simulink model "MPPT"  (R2024a)
settings: Solver=VariableStepAuto  StartTime=0.0  StopTime=0.3  FixedStep=0.02  RelTol=1e-3
libraries: spsSeriesRLCBranchLib x4, spsDiodeLib x2, spsCurrentMeasurementLib x1, spsMosfetLib x1, spsPVArrayLib x1, spsPWMGeneratorDCDCLib x1, spsVoltageMeasurementLib x1, sps_lib x1
settings Model: Creator=ACER  LastModifiedBy=Aswathi Sajeev
settings SolverCC: AlgebraicLoopSolver=TrustRegion
settings DataIOCC: ReturnWorkspaceOutputs=off
settings DebuggingCC: UnconnectedInputMsg=warning  UnconnectedOutputMsg=warning  UnconnectedLineMsg=warning  ArithmeticOperatorsInVariantConditions=warning
settings ModelReferenceCC: EnableRefExpFcnMdlSchedulingChecks=on
settings SFSimCC: SimUseLocalCustomCode=off  CustomCodeUndefinedFunction=UseInterfaceOnly
settings RTWCC: RTWUseLocalCustomCode=off  GPUComputeCapability=3.5

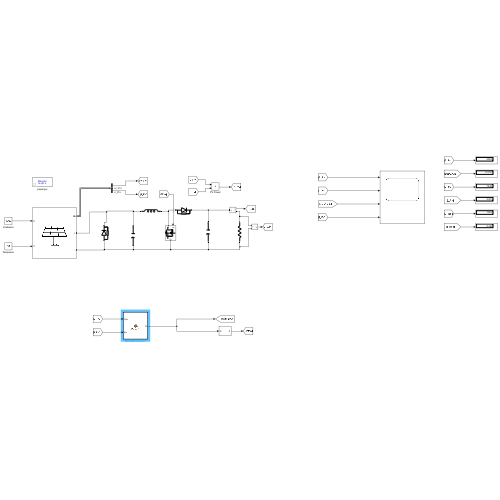
[thumbnail: Simulink's stored preview of the top-level diagram]
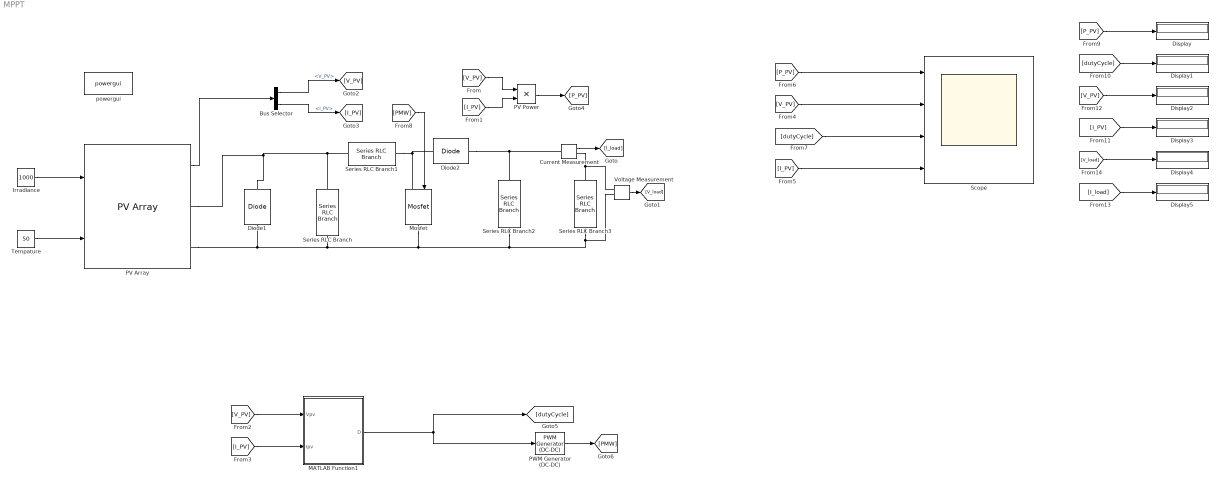
== system MPPT ==
  Bus Selector : BusSelector  OutputSignals=V_PV,I_PV
  Current Measurement : spsCurrentMeasurementLib/Current Measurement  PhasorSimulation=off  OutputType=Complex  PSBequivalent=0
  Diode1 : spsDiodeLib/Diode  Ron=0.001  Lon=0  Vf=0.8  IC=0  UseSnubber=0  Rs=500  Cs=250e-9  Measurements=off
  Diode2 : spsDiodeLib/Diode  Ron=0.001  Lon=0  Vf=0.8  IC=0  UseSnubber=0  Rs=500  Cs=250e-9  Measurements=off
  Display{,1..5} (6 alike) : Display
  Irradiance : Constant  Value=1000
  MATLAB Function1 : MATLAB Function  TreatAsAtomicUnit=on
  Mosfet : spsMosfetLib/Mosfet  Ron=1e-3  Lon=0  Rd=1e-3  Vfd=0  IC=0  Rs=inf  Cs=inf  Measurements=off
  PV Array : spsPVArrayLib/PV Array  Npar=1  Nser=6  PlotType=array @ 1000 W/m2 & specified temperatures  S_vec=[1000 800 400]  Temp_C_vec=[25 50 75]  ModuleName=User-defined  PlotWhenSelected=off  Pm=55.5  Ncell=36  Voc=21.7  Isc=4.8  Vm=15  Im=3.7  beta_Voc_pc=-0.33641  alpha_Isc_pc=0.102  beta_Voc=-0.073001  alpha_Isc=0.004896  IL=5.1461  I0=7.3617e-11  nI=0.95111  Rsh=16.138  Rs=1.1636  RobustModel=off  RobustCellTemperature=313.3991  BAL=off  Tc=1e-6  Tfilter=5e-5
  PV Power : Product
  PWM Generator (DC-DC) : spsPWMGeneratorDCDCLib/PWM Generator (DC-DC)  Fsw=10000  Ts=10e-6
  Scope : Scope  NumInputPorts=4
  Series RLC Branch : spsSeriesRLCBranchLib/Series RLC Branch  LConnTagsString=__new0  RConnTagsString=__new0  BranchType=C  Resistance=1  Inductance=1e-3  SetiL0=off  InitialCurrent=0  Capacitance=470e-6  Setx0=off  InitialVoltage=0  Measurements=None
  Series RLC Branch1 : spsSeriesRLCBranchLib/Series RLC Branch  LConnTagsString=__new0  RConnTagsString=__new0  BranchType=L  Resistance=1  Inductance=1.2e-3  SetiL0=off  InitialCurrent=0  Capacitance=1e-3  Setx0=off  InitialVoltage=0  Measurements=None
  Series RLC Branch2 : spsSeriesRLCBranchLib/Series RLC Branch  LConnTagsString=__new0  RConnTagsString=__new0  BranchType=C  Resistance=1  Inductance=1e-3  SetiL0=off  InitialCurrent=0  Capacitance=47e-6  Setx0=off  InitialVoltage=0  Measurements=None
  Series RLC Branch3 : spsSeriesRLCBranchLib/Series RLC Branch  LConnTagsString=__new0  RConnTagsString=__new0  BranchType=R  Resistance=58  Inductance=1e-3  SetiL0=off  InitialCurrent=0  Capacitance=1e-3  Setx0=off  InitialVoltage=0  Measurements=None
  Tempature : Constant  Value=50
  Voltage Measurement : spsVoltageMeasurementLib/Voltage Measurement  PhasorSimulation=off  OutputType=Complex  PSBequivalent=0
  powergui : sps_lib/powergui  Priority=1  SimulationMode=Discrete  SampleTime=1e-6  frequency=60  Iterations=50  frequencyindice=0  Pbase=100e6  ErrMax=1e-4  UnitsV=kV  UnitsW=MW  buscounter=0  FunctionMessages=off  echomessages=off  EnableUseOfTLC=off  CurrentSourceSwitches=off  DisableSnubberDevices=off  DisableRonSwitches=off  DisableVfSwitches=off  DisplayEquations=off  AutomaticDiscreteSolvers=off  SolverType=Tustin/Backward Euler (TBE)  Interpol=off  ExternalGateDelay=off  methode=off  Ts=100  x0status=blocks  SPID=off  SwTol=0  HookPort=off  NonlinearTolerance=1e-4  nMaxIteration=100  ContinueOnMaxIteration=off  RestoreLinks=warning  ResistiveCurrentMeasurement=off  Frange=[0:2:500]  Ylog=off  Xlog=on  ShowGrid=off  save=off  variable=ZData  structure=0  ZoomFFT=off  StartTime=0.0  cycles=1  DisplayStyle=1  fundamental=60  FreqAxis=off  MaxFrequency=1000  frequencyindicesteady=1  RmsSteady=1  display=off
  wires:
  Irradiance/1 -> PV Array/1
  Tempature/1 -> PV Array/2
  Current Measurement/1 -> [I_load]
  Voltage Measurement/1 -> [V_load]
  PV Array/1 -> Bus Selector/1
  Bus Selector/1 -> [V_PV]  "<V_PV>"
  Bus Selector/2 -> [I_PV]  "<I_PV>"
  [I_PV] -> PV Power/2
  [V_PV] -> PV Power/1
  PV Power/1 -> [P_PV]
  PWM Generator (DC-DC)/1 -> [PMW]
  [V_PV] -> Scope/2
  [P_PV] -> Scope/1
  [dutyCycle] -> Scope/3
  [I_PV] -> Scope/4
  [PMW] -> Mosfet/1
  [P_PV] -> Display/1
  [dutyCycle] -> Display1/1
  [I_PV] -> Display3/1
  [V_PV] -> Display2/1
  [I_load] -> Display5/1
  [V_load] -> Display4/1
  [V_PV] -> MATLAB Function1/1(Vpv)
  [I_PV] -> MATLAB Function1/2(Ipv)
  MATLAB Function1/1(D) -> PWM Generator (DC-DC)/1, [dutyCycle]
  connections:
  PV Array/RConn1 -- Series RLC Branch/LConn1 -- Series RLC Branch1/LConn1 -- Diode1/RConn1
  PV Array/RConn2 -- Voltage Measurement/LConn2 -- Series RLC Branch3/RConn1 -- Series RLC Branch2/RConn1 -- Mosfet/RConn1 -- Series RLC Branch/RConn1 -- Diode1/LConn1
  Diode2/LConn1 -- Series RLC Branch1/RConn1 -- Mosfet/LConn1
  Diode2/RConn1 -- Current Measurement/LConn1 -- Series RLC Branch2/LConn1
  Current Measurement/RConn1 -- Voltage Measurement/LConn1 -- Series RLC Branch3/LConn1

== matlab function MPPT/MATLAB Function1 ==
  settings: updateMethod=DISCRETE
  data: Vpv input; D output; Ipv input
function D = PandO(Vpv,Ipv)

Dinit=0.4;
Dmax=0.9;
Dmin=0.1;
deltaD=20e-6;

persistent Vold Pold Dold;
dataType="double";

if isempty(Vold)
    Vold=0;
    Pold=0;
    Dold=Dinit;
end

P=Vpv*Ipv;
dV=Vpv-Vold;
dP=P-Pold;

if dP ~=0
    if dP<0
        if dV<0
            D = Dold - deltaD;
        else
            D = Dold + deltaD;
        end
    else
        if dV<0
            D = Dold + deltaD;
        else
            D = Dold - deltaD;
        end
    end
else 
    D = Dold;
end
if D>=Dmax || D<=Dmin
    D=Dold;
end

Dold=D;
Vold=Vpv;
Pold=P;
